simulink model "MotorModel_StateSpaceCheck"  (R2015b)
settings: Solver=VariableStepAuto  StartTime=0.0  StopTime=1  RelTol=1e-3
values from neighbouring files (symbols this model uses):
  A_mtr = [ 0 1 0 0 ... (first row only)    [MotorModel_StateSpace.m]    (also in MotorModel_StateSpace_LinearSISO.m = [ 0 1 0)
  B_mtr = [ 0 0 ... (first row only)    [MotorModel_StateSpace.m]    (also in MotorModel_StateSpace_LinearSISO.m = [ 0)
  C_mtr = [ 0 0 1 0 ... (first row only)    [MotorModel_StateSpace.m]    (also in MotorModel_StateSpace_LinearSISO.m = [ 0 1 0 ])
  D_mtr = [ 0 0; 0 0; 0 0 ]    [MotorModel_StateSpace.m]    (also in MotorModel_StateSpace_LinearSISO.m = [ 0; ])
  Vdc = 9.6    [MotorModel_Mabuchi_RS_540.m]    (also in Params.m)
libraries: LocalLib x1
settings Model: Creator=jje  LastModifiedBy=jje

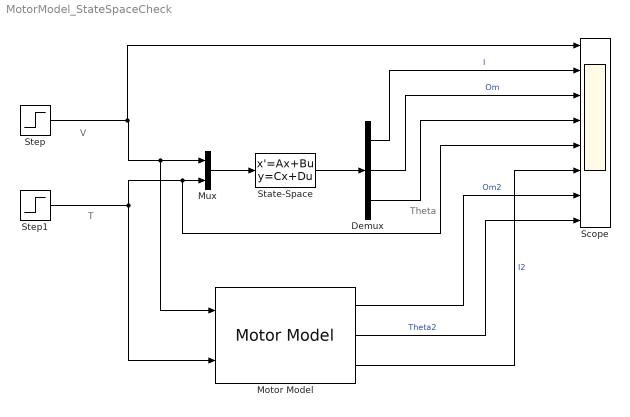
== system MotorModel_StateSpaceCheck ==
  note: Theta
  note: T
  note: V
  Demux : Demux  Outputs=3
  Motor Model : LocalLib/Motor Model
  Mux : Mux  Inputs=2
  Scope : Scope  NumInputPorts=8
  State-Space : StateSpace  A=A_mtr  B=B_mtr  C=C_mtr  D=D_mtr  X0=0
  Step : Step  Time=0.1  After=Vdc  SampleTime=0
  Step1 : Step  Time=0.5  After=-0.1  SampleTime=0
  wires:
  Mux/1 -> State-Space/1
  State-Space/1 -> Demux/1
  Step/1 -> Scope/1, Motor Model/1, Mux/1
  Step1/1 -> Motor Model/2, Scope/5, Mux/2
  Demux/1 -> Scope/2  "I"
  Demux/2 -> Scope/3  "Om"
  Demux/3 -> Scope/4
  Motor Model/1 -> Scope/7  "Om2"
  Motor Model/2 -> Scope/8  "Theta2"
  Motor Model/3 -> Scope/6  "I2"
